simulink model "ControlMode"  (R2020a)
settings: Solver=FixedStepAuto  StartTime=0.0  StopTime=10.0  FixedStep=1e-3  RelTol=1e-3  EnableMultiTasking=on
InitFcn:
  | O_RESPONSE = Simulink.Variant('Response == 1');
  | I_RESPONSE = Simulink.Variant('Response == 2');
  | Response = 1;
settings Model: ExtModeTrigDuration=5  Creator=WinnieTrandinh  LastModifiedBy=WinnieTrandinh
settings OptimizationCC: EnhancedBackFolding=on  PassReuseOutputArgsAs=Individual arguments  ZeroExternalMemoryAtStartup=off  ZeroInternalMemoryAtStartup=off  MaxStackSize=64  OptimizeBlockOrder=speed  DifferentSizesBufferReuse=on  OptimizationCustomize=off  EfficientTunableParamExpr=on
settings DebuggingCC: ParameterTunabilityLossMsg=error
settings HardwareCC: ProdBitPerPointer=32  ProdBitPerSizeT=32  ProdBitPerPtrDiffT=32  ProdLargestAtomicInteger=Long  ProdLargestAtomicFloat=Double  ProdWordSize=32  ProdHWDeviceType=ARM Compatible->ARM Cortex
settings SFSimCC: MATLABDynamicMemAlloc=off
settings RTWCC: SystemTargetFile=ert.tlc  HardwareBoard=NXP FRDM-K64F  TemplateMakefile=ert_default_tmf  Toolchain=GNU Tools for ARM Embedded Processors
settings CodeAppCC: ForceParamTrailComments=on  IgnoreCustomStorageClasses=off  OperatorAnnotations=on  SimulinkDataObjDesc=on  SFDataObjDesc=on  InsertBlockDesc=on

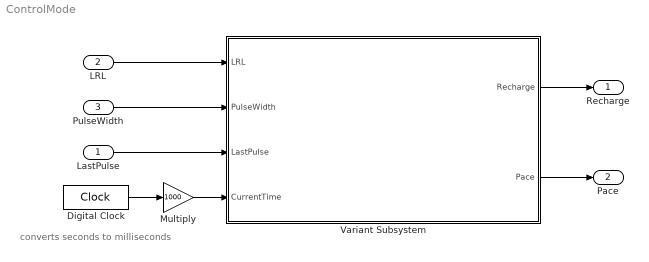
== system ControlMode ==
  note: converts seconds to milliseconds
  LastPulse : Inport
  LRL : Inport  Port=2  Unit=ms
  PulseWidth : Inport  Port=3  Unit=ms
  Digital Clock : DigitalClock  SampleTime=0.001
  Multiply : Gain  Gain=1000
  Variant Subsystem : Subsystem  Variant=on
  Recharge : Outport
  Pace : Outport  Port=2
  wires:
  Digital Clock/1 -> Multiply/1
  Multiply/1 -> Variant Subsystem/4(CurrentTime)
  LastPulse/1 -> Variant Subsystem/3(LastPulse)
  LRL/1 -> Variant Subsystem/1(LRL)
  Variant Subsystem/1(Recharge) -> Recharge/1
  Variant Subsystem/2(Pace) -> Pace/1
  PulseWidth/1 -> Variant Subsystem/2(PulseWidth)

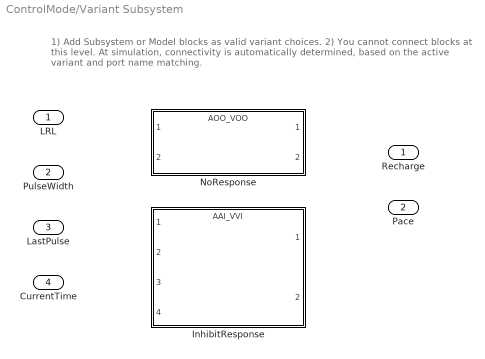
== system ControlMode/Variant Subsystem ==
  note: 1) Add Subsystem or Model blocks as valid variant choices.
      | 2) You cannot connect blocks at this level. At simulation, connectivity is automatically
      | determined, based on the active variant and port name matching.
  LRL : Inport
  PulseWidth : Inport  Port=2
  LastPulse : Inport  Port=3
  CurrentTime : Inport  Port=4
  InhibitResponse : ModelReference  ModelNameDialog=AAI_VVI.slx  SimulationMode=Normal  VariantControl=I_RESPONSE  ModelReferenceVersion=1.6
  NoResponse : ModelReference  ModelNameDialog=AOO_VOO.slx  SimulationMode=Normal  VariantControl=O_RESPONSE  ModelReferenceVersion=1.8
  Recharge : Outport
  Pace : Outport  Port=2
